simulink model "KidApp (1)"  (R2023b)
settings: Solver=FixedStepAuto  StartTime=0.0  StopTime=inf  RelTol=1e-3
undefined symbols (not defined in the file): Fall_Confirmed, Fall_Detected, I_am_Safe, KidApp, Sec, Time_Left_, Your_Current_Speed, Your_istance_From_Origin
libraries: androiduilib x6, simulink x5, androidcommunicationlib x5, androidsensorlib x3, androidaudiovideolib x3
settings Model: Creator=Dell  LastModifiedBy=Dell
settings OptimizationCC: EnhancedBackFolding=on  PassReuseOutputArgsAs=Individual arguments  ZeroExternalMemoryAtStartup=off  ZeroInternalMemoryAtStartup=off  MaxStackSize=64  OptimizeBlockOrder=speed  DifferentSizesBufferReuse=on  OptimizationCustomize=off  EfficientTunableParamExpr=on
settings DebuggingCC: ParameterTunabilityLossMsg=error
settings HardwareCC: ProdBitPerPointer=32  ProdBitPerSizeT=32  ProdBitPerPtrDiffT=32  ProdLargestAtomicInteger=Long  ProdLargestAtomicFloat=Double  ProdWordSize=32  ProdHWDeviceType=ARM Compatible->ARM Cortex  UseEmbeddedCoderFeatures=off  UseSimulinkCoderFeatures=off
settings SFSimCC: MATLABDynamicMemAlloc=off
settings RTWCC: Description=Embedded Coder  SystemTargetFile=ert.tlc  HardwareBoard=Android Device  TLCOptions="-aInlineSetEventsForThisBaseRateFcn=TLC_FALSE -aSuppressMultiTaskScheduler=TLC_FALSE  -aRateBasedStepFcn=0"  TemplateMakefile=ert_default_tmf  RTWVerbose=off  Toolchain=Android SDK/NDK Tools
settings CodeAppCC: ForceParamTrailComments=on  IgnoreCustomStorageClasses=off  OperatorAnnotations=on  SimulinkDataObjDesc=on  SFDataObjDesc=on  InsertBlockDesc=on
settings ERTTargetCC: SupportNonInlinedSFcns=on

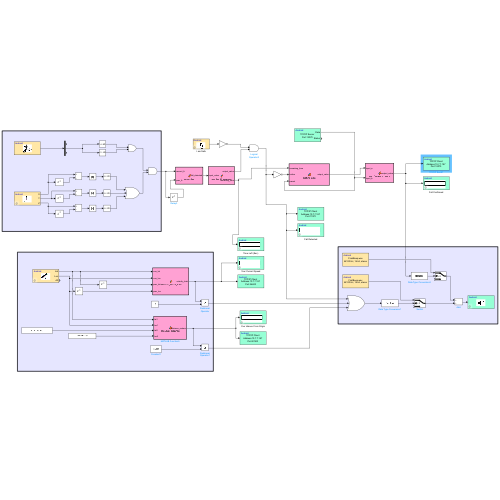
[thumbnail: Simulink's stored preview of the top-level diagram]
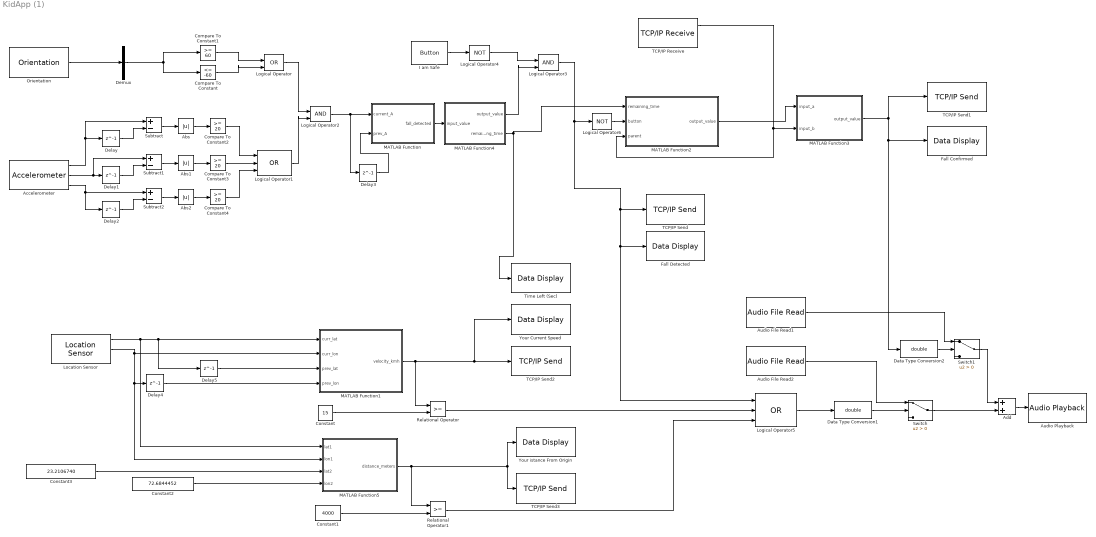
== system KidApp (1) ==
  Abs : Abs  SaturateOnIntegerOverflow=off
  Abs1 : Abs  SaturateOnIntegerOverflow=off
  Abs2 : Abs  SaturateOnIntegerOverflow=off
  Accelerometer : androidsensorlib/Accelerometer  OutputVector=off  SampleTime=0.2  BlockPlatform=Android
  Add : Sum
  Audio File Read1 : androidaudiovideolib/Audio File Read  FileName=C:\Users\Dell\Downloads\FinalBeep.wav  FrameSize=4410
  Audio File Read2 : androidaudiovideolib/Audio File Read  FileName=C:\Users\Dell\Downloads\FirstBeep.wav  FrameSize=4410
  Audio Playback : androidaudiovideolib/Audio Playback  SampleFreq=44100  AudioSamplingFreq=44100  SampleTime=0.1  DeviceStr=0  QueueDuration=0  BlockPlatform=Android
  Compare To Constant : simulink/Logic and Bit Operations/Compare To Constant  relop=<=  const=-60  OutDataTypeStr=boolean
  Compare To Constant1 : simulink/Logic and Bit Operations/Compare To Constant  relop=>=  const=60  OutDataTypeStr=boolean
  Compare To Constant2 : simulink/Logic and Bit Operations/Compare To Constant  relop=>=  const=20  OutDataTypeStr=boolean
  Compare To Constant3 : simulink/Logic and Bit Operations/Compare To Constant  relop=>=  const=20  OutDataTypeStr=boolean
  Compare To Constant4 : simulink/Logic and Bit Operations/Compare To Constant  relop=>=  const=20  OutDataTypeStr=boolean
  Constant : Constant  Value=15
  Constant1 : Constant  Value=4000
  Constant2 : Constant  Value=72.6844452
  Constant3 : Constant  Value=23.2106740
  Data Type Conversion1 : DataTypeConversion  OutDataTypeStr=double  SaturateOnIntegerOverflow=off  RndMeth=Floor
  Data Type Conversion2 : DataTypeConversion  OutDataTypeStr=double  SaturateOnIntegerOverflow=off  RndMeth=Floor
  Delay{,1..5} (6 alike) : Delay  DelayLength=1  InitialCondition=0
  Demux : Demux  Outputs=3
  Fall Confirmed : androiduilib/Data Display  DataDisplayId=KidApp/Fall_Confirmed  Format=Float  Precision=6  SimulateUsing=Code generation  blockPlatform=Android
  Fall Detected : androiduilib/Data Display  DataDisplayId=KidApp/Fall_Detected  Format=Float  Precision=6  SimulateUsing=Code generation  blockPlatform=Android
  I am Safe : androiduilib/Button  ButtonState=Not pressed  ButtonId=KidApp/I_am_Safe  State=off  SampleTime=0.1  BlockPlatform=Android
  Location Sensor : androidsensorlib/Location Sensor  OutputVector=off  SampleTime=4  BlockPlatform=Android
  Logical Operator : Logic  Operator=OR  IconShape=distinctive  AllPortsSameDT=off  OutDataTypeStr=boolean
  Logical Operator1 : Logic  Operator=OR  Inputs=3  IconShape=distinctive  AllPortsSameDT=off  OutDataTypeStr=boolean
  Logical Operator2 : Logic  IconShape=distinctive  AllPortsSameDT=off  OutDataTypeStr=boolean
  Logical Operator3 : Logic  IconShape=distinctive  AllPortsSameDT=off  OutDataTypeStr=boolean
  Logical Operator4 : Logic  Operator=NOT  IconShape=distinctive  AllPortsSameDT=off  OutDataTypeStr=boolean
  Logical Operator5 : Logic  Operator=OR  Inputs=3  IconShape=distinctive  AllPortsSameDT=off  OutDataTypeStr=boolean
  Logical Operator6 : Logic  Operator=NOT  IconShape=distinctive  AllPortsSameDT=off  OutDataTypeStr=boolean
  MATLAB Function : MATLAB Function  TreatAsAtomicUnit=on
  MATLAB Function1 : MATLAB Function  TreatAsAtomicUnit=on
  MATLAB Function2 : MATLAB Function  TreatAsAtomicUnit=on
  MATLAB Function3 : MATLAB Function  TreatAsAtomicUnit=on
  MATLAB Function4 : MATLAB Function  TreatAsAtomicUnit=on
  MATLAB Function5 : MATLAB Function  TreatAsAtomicUnit=on
  Orientation : androidsensorlib/Orientation  SampleTime=0.2
  Relational Operator : RelationalOperator  OutDataTypeStr=boolean  RndMeth=Simplest  InputSameDT=off
  Relational Operator1 : RelationalOperator  OutDataTypeStr=boolean  RndMeth=Simplest  InputSameDT=off
  Subtract : Sum  Inputs=+-
  Subtract1 : Sum  Inputs=+-
  Subtract2 : Sum  Inputs=+-
  Switch : Switch  Criteria=u2 > Threshold  SaturateOnIntegerOverflow=off  InputSameDT=off
  Switch1 : Switch  Criteria=u2 > Threshold  SaturateOnIntegerOverflow=off  InputSameDT=off
  TCP/IP Receive : androidcommunicationlib/TCP//IP Receive  TCPReceiveId=KidApp/TCP//IP_Receive  Mode_=Server  LocalServerPort_=13070  RemoteAddr_=127.0.0.1  RemoteServerPort_=25000  DataType_=boolean  DataSize_=1  SampleTime_=0.1  ClientPortBindingSelection_=off  ClientPortToBind_=35000  BlockingMode_=off  BlockTimeout_=0.1
  TCP/IP Send : androidcommunicationlib/TCP//IP Send  TCPSendId=KidApp/TCP//IP_Send  Mode_=Client  LocalServerPort_=25000  RemoteAddr_=10.7.7.187  RemoteServerPort_=11070  ClientPortBindingSelection_=off  ClientPortToBind_=35000  BlockingMode_=off  BlockTimeout_=0.1
  TCP/IP Send1 : androidcommunicationlib/TCP//IP Send  TCPSendId=KidApp/TCP//IP_Send1  Mode_=Client  LocalServerPort_=25000  RemoteAddr_=10.7.7.187  RemoteServerPort_=12070  ClientPortBindingSelection_=off  ClientPortToBind_=35000  BlockingMode_=off  BlockTimeout_=0.1
  TCP/IP Send2 : androidcommunicationlib/TCP//IP Send  TCPSendId=KidApp/TCP//IP_Send2  Mode_=Client  LocalServerPort_=25000  RemoteAddr_=10.7.7.187  RemoteServerPort_=26600  ClientPortBindingSelection_=off  ClientPortToBind_=35000  BlockingMode_=off  BlockTimeout_=0.1
  TCP/IP Send3 : androidcommunicationlib/TCP//IP Send  TCPSendId=KidApp/TCP//IP_Send3  Mode_=Client  LocalServerPort_=25000  RemoteAddr_=10.7.7.187  RemoteServerPort_=27600  ClientPortBindingSelection_=off  ClientPortToBind_=35000  BlockingMode_=off  BlockTimeout_=0.1
  Time Left (Sec) : androiduilib/Data Display  DataDisplayId=KidApp/Time_Left_(Sec)  Format=Float  Precision=6  SimulateUsing=Code generation  blockPlatform=Android
  Your Current Speed : androiduilib/Data Display  DataDisplayId=KidApp/Your_Current_Speed  Format=Float  Precision=6  SimulateUsing=Code generation  blockPlatform=Android
  Your istance From Origin : androiduilib/Data Display  DataDisplayId=KidApp/Your_istance_From_Origin  Format=Float  Precision=6  SimulateUsing=Code generation  blockPlatform=Android
  wires:
  Orientation/1 -> Demux/1
  Demux/2 -> Compare To Constant/1, Compare To Constant1/1
  Accelerometer/1 -> Subtract/1, Delay/1
  Compare To Constant1/1 -> Logical Operator/1
  Compare To Constant/1 -> Logical Operator/2
  Delay/1 -> Subtract/2
  Subtract/1 -> Abs/1
  Abs/1 -> Compare To Constant2/1
  Delay1/1 -> Subtract1/2
  Abs1/1 -> Compare To Constant3/1
  Subtract1/1 -> Abs1/1
  Accelerometer/2 -> Subtract1/1, Delay1/1
  Delay2/1 -> Subtract2/2
  Abs2/1 -> Compare To Constant4/1
  Subtract2/1 -> Abs2/1
  Accelerometer/3 -> Subtract2/1, Delay2/1
  Compare To Constant3/1 -> Logical Operator1/2
  Compare To Constant2/1 -> Logical Operator1/1
  Compare To Constant4/1 -> Logical Operator1/3
  Logical Operator/1 -> Logical Operator2/1
  Logical Operator1/1 -> Logical Operator2/2
  Logical Operator2/1 -> Delay3/1, MATLAB Function/1(current_A)
  Delay3/1 -> MATLAB Function/2(prev_A)
  I am Safe/1 -> Logical Operator4/1
  MATLAB Function/1(fall_detected) -> MATLAB Function4/1(input_value)
  Logical Operator4/1 -> Logical Operator3/1
  Logical Operator3/1 -> Logical Operator5/1, Fall Detected/1, TCP/IP Send/1, Logical Operator6/1
  TCP/IP Receive/1 -> MATLAB Function2/3(parent), MATLAB Function3/2(input_b)
  MATLAB Function4/2(remaining_time) -> MATLAB Function2/1(remaining_time), Time Left (Sec)/1
  MATLAB Function4/1(output_value) -> Logical Operator3/2
  MATLAB Function3/1(output_value) -> Fall Confirmed/1, Data Type Conversion2/1, TCP/IP Send1/1
  MATLAB Function2/1(output_value) -> MATLAB Function3/1(input_a)
  Delay4/1 -> MATLAB Function1/4(prev_lon)
  MATLAB Function5/1(distance_meters) -> Relational Operator1/1, TCP/IP Send3/1, Your istance From Origin/1
  Constant2/1 -> MATLAB Function5/4(lon2)
  Constant3/1 -> MATLAB Function5/3(lat2)
  Constant1/1 -> Relational Operator1/2
  MATLAB Function1/1(velocity_kmh) -> Your Current Speed/1, TCP/IP Send2/1, Relational Operator/1
  Delay5/1 -> MATLAB Function1/3(prev_lat)
  Constant/1 -> Relational Operator/2
  Location Sensor/1 -> MATLAB Function1/1(curr_lat), Delay5/1, MATLAB Function5/1(lat1)
  Location Sensor/2 -> MATLAB Function5/2(lon1), Delay4/1, MATLAB Function1/2(curr_lon)
  Relational Operator/1 -> Logical Operator5/2
  Relational Operator1/1 -> Logical Operator5/3
  Logical Operator5/1 -> Data Type Conversion1/1
  Audio File Read2/1 -> Switch/1
  Data Type Conversion1/1 -> Switch/2
  Data Type Conversion2/1 -> Switch1/2
  Audio File Read1/1 -> Switch1/1
  Switch/1 -> Add/2
  Switch1/1 -> Add/1
  Add/1 -> Audio Playback/1
  Logical Operator6/1 -> MATLAB Function2/2(button)

== matlab function KidApp (1)/MATLAB Function1 ==
  data: curr_lat input; velocity_kmh output; curr_lon input; prev_lat input; prev_lon input
function velocity_kmh = calculate_speed_kmh(curr_lat, curr_lon, prev_lat, prev_lon)
    % Radius of the Earth in kilometers
    R = 6371.0;

    % Convert latitude and longitude from degrees to radians
    curr_lat = deg2rad(curr_lat);
    curr_lon = deg2rad(curr_lon);
    prev_lat = deg2rad(prev_lat);
    prev_lon = deg2rad(prev_lon);

    % Haversine formula to calculate distance
    d = 2 * R * asin(sqrt(sin((curr_lat - prev_lat) / 2)^2 + cos(prev_lat) * cos(curr_lat) * sin((curr_lon - prev_lon) / 2)^2));

    % Calculate speed in km/h
    time_difference_hours = 4 / 3600;  % 1 second time difference in hours
    velocity_kmh = d / time_difference_hours;  % Speed in km/h
end

== matlab function KidApp (1)/MATLAB Function ==
  data: current_A input; fall_detected output; prev_A input
function fall_detected = detect_fall(current_A, prev_A)
    % Check for a change in A (current A is true and prev A is false)

    if current_A && ~prev_A
        fallDetectedState = true;
    else
        fallDetectedState = false;
    end
    
    fall_detected = fallDetectedState;
end

== matlab function KidApp (1)/MATLAB Function2 ==
  data: remaining_time input; output_value output; button input; parent input
function output_value = custom_logic(remaining_time, button, parent)

    persistent output_state;
    
    % Initialize output_state to false if it's not already defined.
    if isempty(output_state)
        output_state = false;
    end
    
    % Check if parent is true, and if so, reset the output and return false.
    if parent
        output_state = false;
        output_value = false;
        return;
    end
    
    % Check if remaining_time is greater than 0.1 and button is true.
    if 0.5 > remaining_time && remaining_time > 0.1 && ~button
        % If the conditions are met, set the output to true.
        output_state = true;
    else
        % If the conditions are not met, maintain the previous output state.
    end
    
    % Output the current state.
    output_value = output_state;
end

== matlab function KidApp (1)/MATLAB Function3 ==
  data: input_a input; output_value output; input_b input
function output_value = true_forever_when_a(input_a, input_b)
    % Define a persistent variable to store the state
    persistent is_output_true
    is_output_true = false;
    
    % Initialize the state if it's not already initialized
    if isempty(is_output_true)
        is_output_true = false;
    end
    
    % Update the state based on input
    if input_a
        is_output_true = true;
    end
    
    if input_b
        is_output_true = false;
    end
    
    % Output the current state
    output_value = is_output_true;
end

== matlab function KidApp (1)/MATLAB Function4 ==
  data: input_value input; output_value output; remaining_time output
function [output_value, remaining_time] = true_for_5_seconds(input_value)
    % Define a persistent variable to store the timestamp when input becomes true
    persistent true_timestamp
    
    % Initialize the persistent variable if input becomes true
    if input_value
        true_timestamp = tic;  % Record the current time
    end
    
    % Check if 5 seconds have passed since the input became true
    if ~isempty(true_timestamp) && toc(true_timestamp) <= 5
        output_value = true;
        remaining_time = 5 - toc(true_timestamp);
    else
        % Reset the persistent variables and output 'false'
        output_value = false;
        remaining_time = 0;
    end
end

== matlab function KidApp (1)/MATLAB Function5 ==
  data: lat1 input; distance_meters output; lon1 input; lat2 input; lon2 input
function distance_meters = calculate_distance(lat1, lon1, lat2, lon2)
    % Radius of the Earth in meters
    R = 6371000;  % Mean radius of the Earth in meters

    % Convert latitude and longitude from degrees to radians
    lat1 = deg2rad(lat1);
    lon1 = deg2rad(lon1);
    lat2 = deg2rad(lat2);
    lon2 = deg2rad(lon2);

    % Haversine formula to calculate distance
    dlat = lat2 - lat1;
    dlon = lon2 - lon1;

    a = sin(dlat/2)^2 + cos(lat1) * cos(lat2) * sin(dlon/2)^2;
    c = 2 * atan2(sqrt(a), sqrt(1 - a));

    % Calculate distance in meters
    distance_meters = R * c;
end
